simulink library "UtilityLibrary"  (R2021a)
settings: Solver=VariableStepAuto  StartTime=0.0  StopTime=10.0  RelTol=1e-3
settings Model: Creator=phill  LastModifiedBy=phill

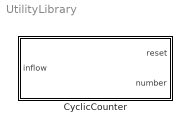
== system UtilityLibrary ==
  CyclicCounter : Subsystem  mask{resetThreshold=1}
      mask prompts: resetThreshold "reset threshold"
      mask Display:
      | disp('flow ctr \n\n');
      | disp(['resets at x = ', get_param(gcb,'resetThreshold')])

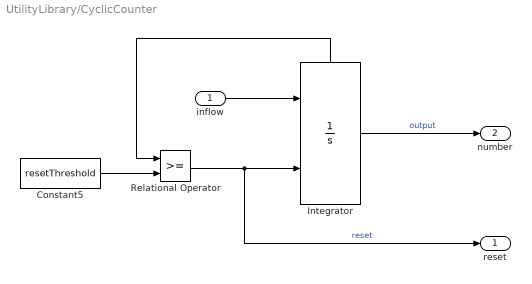
== system UtilityLibrary/CyclicCounter ==
  inflow : Inport
  Constant5 : Constant  Value=resetThreshold
  Integrator : Integrator  ExternalReset=rising  LimitOutput=on  UpperSaturationLimit=resetThreshold  LowerSaturationLimit=0  ShowStatePort=on
  Relational Operator : RelationalOperator  OutDataTypeStr=boolean  RndMeth=Simplest
  reset : Outport
  number : Outport  Port=2
  wires:
  Constant5/1 -> Relational Operator/2
  Integrator/1 -> number/1  "output"
  inflow/1 -> Integrator/1
  Relational Operator/1 -> Integrator/2, reset/1  "reset"
  Integrator/State -> Relational Operator/1
